simulink model "ADM1"  (R2019b)
settings: Solver=VariableStepAuto  StartTime=0.0  StopTime=100.0  RelTol=1e-3
undefined symbols (not defined in the file or in its folder): initial, parameters, system
settings Model: Creator=sweinrich  LastModifiedBy=sweinrich

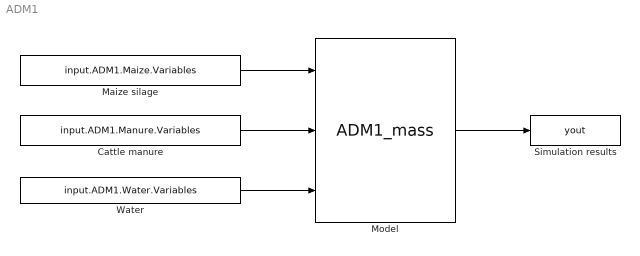
== system ADM1 ==
  Cattle manure : FromWorkspace  VariableName=input.ADM1.Manure.Variables  SampleTime=0  Interpolate=off  OutputAfterFinalValue=Holding final value
  Maize silage : FromWorkspace  VariableName=input.ADM1.Maize.Variables  SampleTime=0  Interpolate=off  OutputAfterFinalValue=Holding final value
  Model : S-Function  FunctionName=ADM1_mass  Parameters=initial.ADM1.Variables',parameters.ADM1.Variables,system.Variables,3,0  SFunctionDeploymentMode=off  EnableBusSupport=off
  Simulation results : ToWorkspace  VariableName=yout  SampleTime=-1
      settings: Save2DSignal=2-D array (concatenate along first dimension)
  Water : FromWorkspace  VariableName=input.ADM1.Water.Variables  SampleTime=0  Interpolate=off  OutputAfterFinalValue=Holding final value
  wires:
  Model/1 -> Simulation results/1
  Water/1 -> Model/3
  Cattle manure/1 -> Model/2
  Maize silage/1 -> Model/1
